simulink model "Ex_1_Passive_Low_Pass_Filter_Simplified"  (R2020a)
settings: Solver=FixedStepAuto  StartTime=0.0  StopTime=0.005  FixedStep=0.000001  RelTol=1e-3
libraries: powerlib_meascontrol x1
settings Model: Creator=alexr  LastModifiedBy=alexr

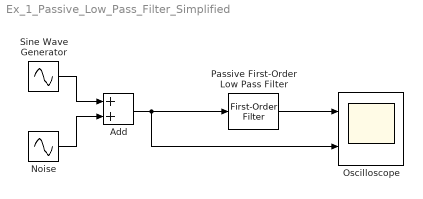
== system Ex_1_Passive_Low_Pass_Filter_Simplified ==
  Add : Sum
  Noise : Sin  Amplitude=0.5  Frequency=2*pi*20000  SampleTime=0
  Oscilloscope : Scope  NumInputPorts=2
  Passive First-Order Low Pass Filter : powerlib_meascontrol/Filters/First-Order Filter  FilterType=Lowpass  Tc=1000*0.1*10^-6  Ts=0  Initialize=off  Vac_Init=[0, 0, 60]  Vdc_Init=0  PlotResponse=off  FreqRange="[0,  10000,  1]"
  Sine Wave Generator : Sin  Amplitude=3  Frequency=2*pi*200  SampleTime=0
  wires:
  Passive First-Order Low Pass Filter/1 -> Oscilloscope/1
  Sine Wave Generator/1 -> Add/1
  Noise/1 -> Add/2
  Add/1 -> Oscilloscope/2, Passive First-Order Low Pass Filter/1
